simulink model "MySusp_Buffer_RTW"  (Simulink 9.1)
settings: Solver=ode1  StartTime=0.0  StopTime=inf  FixedStep=0.001  RelTol=1e-3
PreLoadFcn:
  | vehicle = 'Car'; if ~length(which('cmself')), cmenv; end
  | MySusp_Buffer_RTW_bus
  | MySusp_Buffer_RTW_params
InitFcn:
  | vehicle = 'Car'; if ~length(which('cmself')), cmenv; end
  | MySusp_Buffer_RTW_bus
undefined symbols (not defined in the file): l0_Pull, l0_Push, Stiffness_Pull, Stiffness_Push
Description:
  | CarMaker Plug-in Model Target
settings Model: SuppressorTable=22 serialization::archive 11 0 6 0 0 0 1 0  Creator=ml  LastModifiedBy=ml
settings DataIOCC: SaveFormat=Dataset
settings OptimizationCC: LifeSpan=auto
settings DebuggingCC: UnderspecifiedInitializationDetection=Simplified  MergeDetectMultiDrivingBlocksExec=error  SFUnexpectedBacktrackingDiag=error  SFNoUnconditionalDefaultTransitionDiag=error  SFExecutionAtInitializationDiag=warning
settings HardwareCC: ProdBitPerPointer=64  ProdBitPerSizeT=64  ProdBitPerPtrDiffT=64  ProdLargestAtomicFloat=Float  ProdIntDivRoundTo=Zero  ProdEndianess=LittleEndian  ProdWordSize=64  ProdHWDeviceType=Intel->x86-64 (Windows64)
settings ModelReferenceCC: PropagateSignalLabelsOutOfModel=on
settings RTWCC: SystemTargetFile=CarMaker.tlc  TemplateMakefile=CarMaker_unix-win64.tmf  Description=CarMaker Plug-in Model Target
settings CodeAppCC: MaxIdLength=127
settings STFCustomTargetCC: TargetLangStandard=C99 (ISO)  CombineOutputUpdateFcns=on  MultiInstanceERTCode=on  CodeInterfacePackaging=Reusable function  GRTInterface=off  GenerateAllocFcn=on  SystemTargetFile=CarMaker.tlc
settings GRTTargetCC: TargetLangStandard=C99 (ISO)  ParMdlRefBuildCompliant=off  CompOptLevelCompliant=off  ConcurrentExecutionCompliant=off  CombineOutputUpdateFcns=on  MatFileLogging=off  MultiInstanceERTCode=on  CodeInterfacePackaging=Reusable function  CPPClassGenCompliant=off  GRTInterface=off  GenerateAllocFcn=on  UseToolchainInfoCompliant=off  RTWCAPISignals=on  RTWCAPIParams=on  RTWCAPIStates=on
settings CustomProperty: DataType=string
settings EnumStrPairs: String=Car
settings ConfigComp: CovMetricSettings=dwe  CovHtmlReporting=off  CovSaveCumulativeToWorkspaceVar=off  CovSaveSingleToWorkspaceVar=off  CovExternalEMLEnable=on

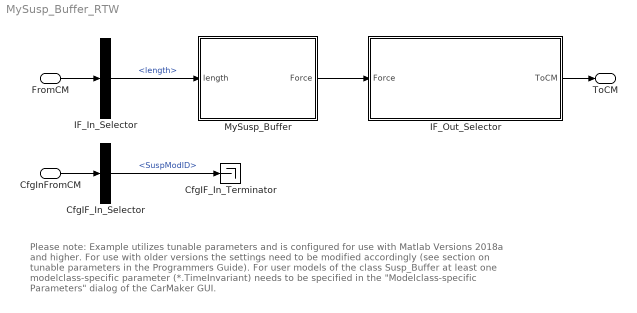
== system MySusp_Buffer_RTW ==
  note: Please note: Example utilizes tunable parameters and is configured for use with Matlab Versions 2018a and higher.
      | For use with older versions the settings need to be modified accordingly (see section on tunable parameters in the Programmers Guide).
      |
      | For user models of the class Susp_Buffer at least one modelclass-specific parameter (*.TimeInvariant) needs to be specified in the
      | "Modelclass-specific Parameters" dialog of the CarMaker GUI.
  FromCM : Inport  OutDataTypeStr=Bus: cmSusp_BufferIn
  CfgInFromCM : Inport  Port=2  OutDataTypeStr=Bus: cmSusp_BufferCfgIn
  CfgIF_In_Selector : BusSelector  OutputSignals=SuspModID
  CfgIF_In_Terminator : Terminator
  IF_In_Selector : BusSelector  OutputSignals=length
  IF_Out_Selector : Subsystem  mask(Signal Selection){}
      mask help: Signal Selection Block
      settings: OpenFcn=cmSignalSelect('SignalSelection_CB',gcb)
  MySusp_Buffer : Subsystem
  ToCM : Outport  OutDataTypeStr=Bus: cmSusp_BufferOut
  wires:
  FromCM/1 -> IF_In_Selector/1
  IF_Out_Selector/1(ToCM) -> ToCM/1
  CfgInFromCM/1 -> CfgIF_In_Selector/1
  CfgIF_In_Selector/1 -> CfgIF_In_Terminator/1  "<SuspModID>"
  IF_In_Selector/1 -> MySusp_Buffer/1(length)  "<length>"
  MySusp_Buffer/1(Force) -> IF_Out_Selector/1(Force)

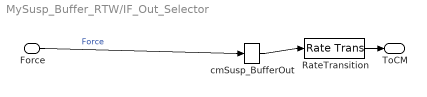
== system MySusp_Buffer_RTW/IF_Out_Selector ==
  Force : Inport
  RateTransition : RateTransition  OutPortSampleTime=str2num(get_param(bdroot,'FixedStep'))
  cmSusp_BufferOut : BusCreator  Inputs=1
  ToCM : Outport
  wires:
  RateTransition/1 -> ToCM/1
  cmSusp_BufferOut/1 -> RateTransition/1
  Force/1 -> cmSusp_BufferOut/1  "Force"

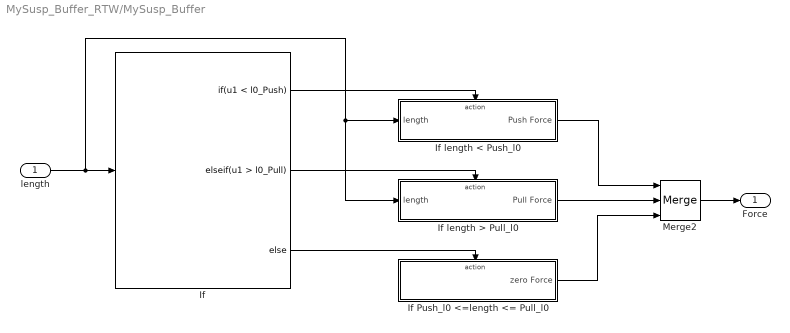
== system MySusp_Buffer_RTW/MySusp_Buffer ==
  length : Inport
  If : If  IfExpression=u1 < l0_Push  ElseIfExpressions=u1 > l0_Pull
  "If Push_l0 <=length <= Pull_l0 " : Subsystem  TreatAsAtomicUnit=on
  If length < Push_l0 : Subsystem  TreatAsAtomicUnit=on
  If length > Pull_l0 : Subsystem  TreatAsAtomicUnit=on
  Merge2 : Merge  Inputs=3
  Force : Outport
  wires:
  length/1 -> If length > Pull_l0/1(length), If length < Push_l0/1(length), If/1
  If/3 -> "If Push_l0 <=length <= Pull_l0 "/Action
  If/2 -> If length > Pull_l0/Action
  If/1 -> If length < Push_l0/Action
  If length < Push_l0/1(Push Force) -> Merge2/1
  "If Push_l0 <=length <= Pull_l0 "/1(zero Force) -> Merge2/3
  If length > Pull_l0/1(Pull Force) -> Merge2/2
  Merge2/1 -> Force/1

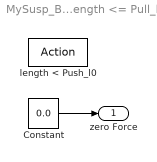
== system MySusp_Buffer_RTW/MySusp_Buffer/If Push_l0 <=length <= Pull_l0  ==
  length < Push_l0 : ActionPort  ActionType=else
  Constant : Constant  Value=0.0
  zero Force : Outport  InitialOutput=0
  wires:
  Constant/1 -> zero Force/1

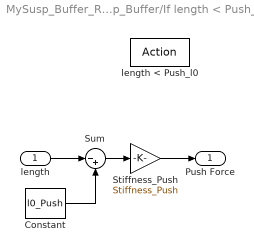
== system MySusp_Buffer_RTW/MySusp_Buffer/If length < Push_l0 ==
  length : Inport
  length < Push_l0 : ActionPort  ActionType=then
  Constant : Constant  Value=l0_Push
  Stiffness_Push : Gain  Gain=Stiffness_Push
  Sum : Sum  Inputs=|-+
  Push Force : Outport  InitialOutput=0
  wires:
  length/1 -> Sum/1
  Stiffness_Push/1 -> Push Force/1
  Sum/1 -> Stiffness_Push/1
  Constant/1 -> Sum/2

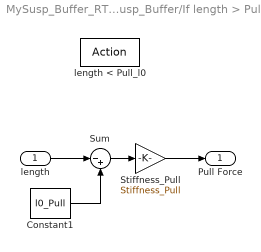
== system MySusp_Buffer_RTW/MySusp_Buffer/If length > Pull_l0 ==
  length : Inport
  length < Pull_l0 : ActionPort  ActionType=elseif
  Constant1 : Constant  Value=l0_Pull
  "Stiffness_Pull " : Gain  Gain=Stiffness_Pull
  Sum : Sum  Inputs=|-+
  Pull Force : Outport  InitialOutput=0
  wires:
  "Stiffness_Pull "/1 -> Pull Force/1
  Sum/1 -> "Stiffness_Pull "/1
  Constant1/1 -> Sum/2
  length/1 -> Sum/1
